simulink model "tp1_cdm"  (R2018b)
settings: Solver=FixedStepAuto  StartTime=0.0  StopTime=6  RelTol=1e-3
settings Model: Creator=e12210406  LastModifiedBy=e12210406

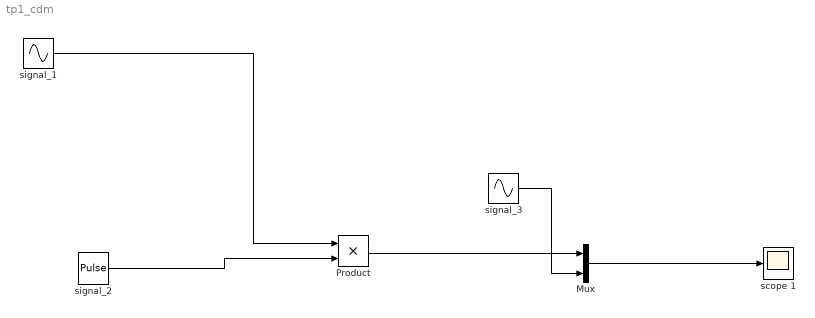
== system tp1_cdm ==
  Mux : Mux  Inputs=2
  Product : Product
  "scope 1 " : Scope
  signal_1 : Sin  Frequency=2080  SampleTime=0
  "signal_2 " : DiscretePulseGenerator  PulseType=Time based  Period=2*pi/1000  PulseWidth=0.1
  signal_3 : Sin  Frequency=80  SampleTime=0
  wires:
  signal_1/1 -> Product/1
  "signal_2 "/1 -> Product/2
  Product/1 -> Mux/1
  Mux/1 -> "scope 1 "/1
  signal_3/1 -> Mux/2
